simulink model "nonlinear_system"  (R2023b)
settings: Solver=VariableStepAuto  StartTime=0.0  StopTime=10  RelTol=1e-3
values from neighbouring files (symbols this model uses):
  Bl = 0    [collaborative_class_main.m]    (also in n0_collaborative_class_main.m; svc_robot.m)
  Bm = 0.015    [collaborative_class_main.m]    (also in n0_collaborative_class_main.m; svc_robot.m)
  g = 9.81    [collaborative_class_main.m]    (also in n0_collaborative_class_main.m; svc_robot.m)
  Jl = 4e-4    (= 0.0004)    [collaborative_class_main.m]    (also in n0_collaborative_class_main.m; svc_robot.m)
  Jm = 4e-4    (= 0.0004)    [collaborative_class_main.m]    (also in n0_collaborative_class_main.m; svc_robot.m)
  k = 0.8    [collaborative_class_main.m]    (also in n0_collaborative_class_main.m; svc_robot.m)
  K_lqeta = K_lqe(:, 5)    [collaborative_class_main.m]    (also in n0_collaborative_class_main.m = K_lq_ext(:,5))
  K_lqx = K_lqe(:,1:4)    [collaborative_class_main.m]    (also in n0_collaborative_class_main.m = K_lq_ext(:,1:4))
  Kv = -K_ext(1, 5)    [collaborative_class_main.m]    (also in n0_collaborative_class_main.m)
  Kx = -K_ext(1, 1:4)    [collaborative_class_main.m]    (also in n0_collaborative_class_main.m)
  l = 0.3    [collaborative_class_main.m]    (also in n0_collaborative_class_main.m; svc_robot.m)
  m = 0.3    [collaborative_class_main.m]    (also in n0_collaborative_class_main.m; svc_robot.m)
  u_bar = m*g*l*cos(x2_bar)    [collaborative_class_main.m]    (also in n0_collaborative_class_main.m; svc_robot.m)
  x_0 = x_bar+0.01    [collaborative_class_main.m]
  x_bar = [x1_bar x2_bar x3_bar x4_bar]    [collaborative_class_main.m]    (also in n0_collaborative_class_main.m; svc_robot.m = [x1_bar x2_bar x3_bar x4_bar]')
settings Model: Creator=alexz  LastModifiedBy=teoma

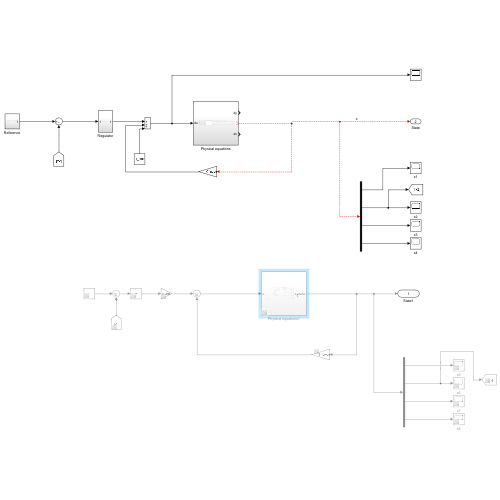
[thumbnail: Simulink's stored preview of the top-level diagram]
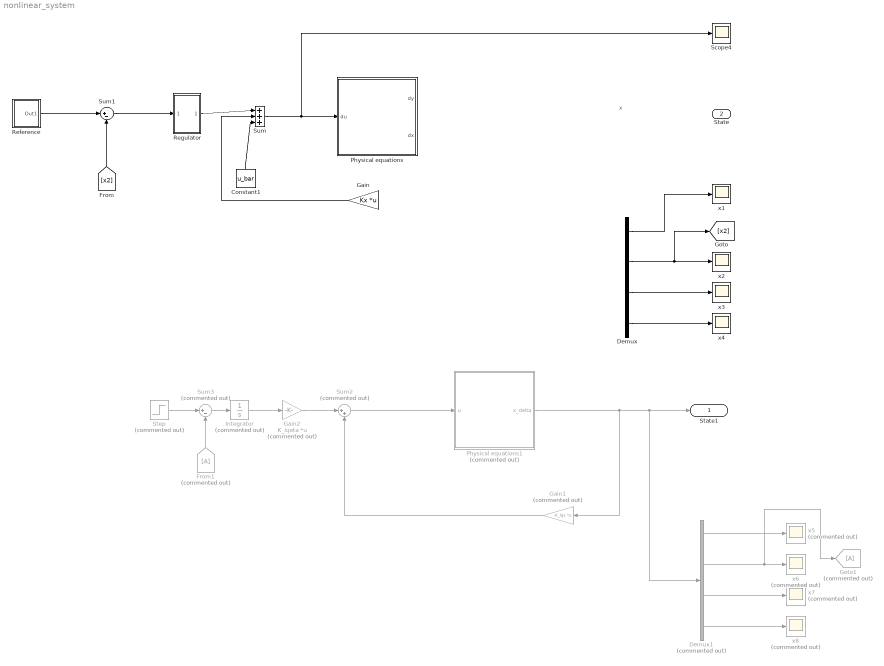
== system nonlinear_system ==
  note: x
  Constant1 : Constant  Value=u_bar
  Demux : Demux
  Demux1 : Demux  Commented=on
  From1 : From  Commented=on
  Gain : Gain  Gain=Kx  Multiplication=Matrix(K*u) (u vector)
  Gain1 : Gain  Commented=on  Gain=-K_lqx  Multiplication=Matrix(K*u) (u vector)
  Gain2 : Gain  Commented=on  Gain=K_lqeta  Multiplication=Matrix(K*u) (u vector)
  Goto1 : Goto  Commented=on
  Integrator : Integrator  Commented=on
  Physical equations : Subsystem
  Physical equations1 : Subsystem  Commented=on
  Reference : Subsystem
  Regulator : Subsystem
  Scope4 : Scope
  Step : Step  Commented=on  SampleTime=0
  Sum : Sum  Inputs=|+++
  Sum1 : Sum  Inputs=|+-
  Sum2 : Sum  Commented=on  Inputs=|++
  Sum3 : Sum  Commented=on  Inputs=|+-
  x{1..4} (4 alike) : Scope
  x{5..8} (4 alike) : Scope  Commented=on
  State1 : Outport
  State : Outport  Port=2
  wires:
  Sum1/1 -> Regulator/1(In1)
  [x2] -> Sum1/2
  Regulator/1(Out1) -> Sum/1
  ? -> Demux/1, State/1, Gain/1
  Gain/1 -> Sum/2
  Sum/1 -> Physical equations/1(du), Scope4/1
  Demux/1 -> x1/1
  Demux/4 -> x4/1
  Demux/3 -> x3/1
  Demux/2 -> [x2], x2/1
  Reference/1(Out1) -> Sum1/1
  Constant1/1 -> Sum/3
  Physical equations1/1(x_delta) -> Gain1/1, Demux1/1, State1/1
  Sum2/1 -> Physical equations1/1(u)
  Gain1/1 -> Sum2/2
  Demux1/1 -> x5/1
  Demux1/4 -> x8/1
  Demux1/3 -> x7/1
  Demux1/2 -> Goto1/1, x6/1
  Sum3/1 -> Integrator/1
  From1/1 -> Sum3/2
  Gain2/1 -> Sum2/1
  Integrator/1 -> Gain2/1
  Step/1 -> Sum3/1

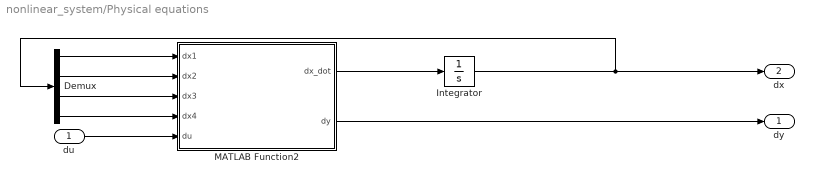
== system nonlinear_system/Physical equations ==
  du : Inport
  Demux : Demux
  Integrator : Integrator  InitialCondition=[0;0;0;0]+1
  MATLAB Function2 : MATLAB Function  TreatAsAtomicUnit=on
  dy : Outport
  dx : Outport  Port=2
  wires:
  MATLAB Function2/2(dy) -> dy/1
  MATLAB Function2/1(dx_dot) -> Integrator/1
  du/1 -> MATLAB Function2/5(du)
  Demux/3 -> MATLAB Function2/3(dx3)
  Demux/2 -> MATLAB Function2/2(dx2)
  Demux/1 -> MATLAB Function2/1(dx1)
  Integrator/1 -> Demux/1, dx/1
  Demux/4 -> MATLAB Function2/4(dx4)

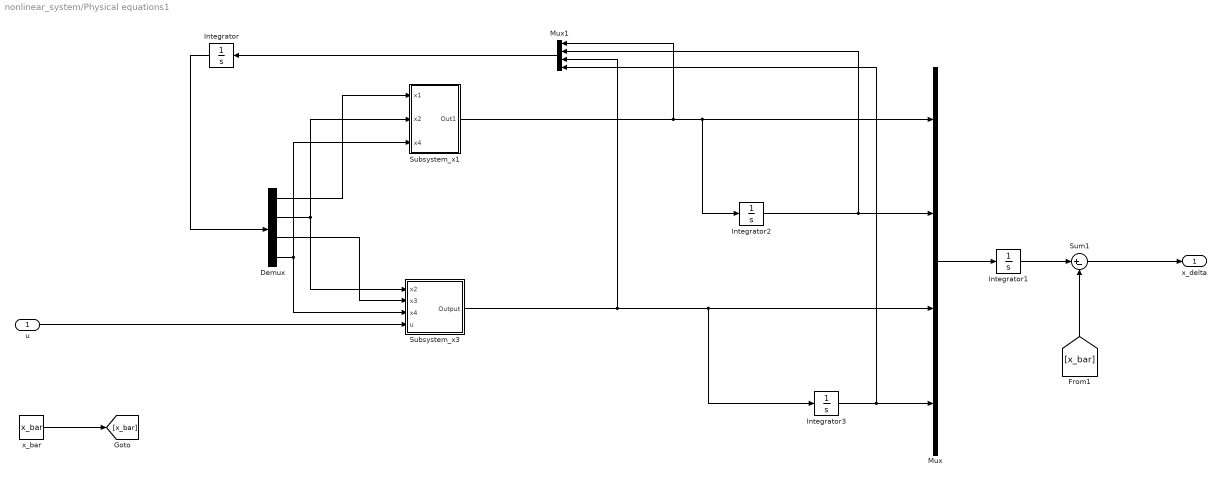
== system nonlinear_system/Physical equations1 ==
  u : Inport
  Demux : Demux
  Integrator : Integrator  InitialCondition=x_0
  Integrator1 : Integrator
  Integrator2 : Integrator
  Integrator3 : Integrator
  Mux : Mux
  Mux1 : Mux
  Subsystem_x1 : Subsystem
  Subsystem_x3 : Subsystem
  Sum1 : Sum  Inputs=|+-
  x_bar : Constant  Value=x_bar
  x_delta : Outport
  wires:
  u/1 -> Subsystem_x3/4(u)
  Integrator/1 -> Demux/1
  x_bar/1 -> [x_bar]
  Mux1/1 -> Integrator/1
  Mux/1 -> Integrator1/1
  Demux/1 -> Subsystem_x1/1(x1)
  Demux/2 -> Subsystem_x3/1(x2), Subsystem_x1/2(x2)
  Demux/3 -> Subsystem_x3/2(x3)
  Subsystem_x3/1(Output) -> Mux1/3, Integrator3/1, Mux/3
  Demux/4 -> Subsystem_x3/3(x4), Subsystem_x1/3(x4)
  Subsystem_x1/1(Out1) -> Mux1/1, Integrator2/1, Mux/1
  Integrator2/1 -> Mux1/2, Mux/2
  Integrator3/1 -> Mux1/4, Mux/4
  [x_bar] -> Sum1/2
  Integrator1/1 -> Sum1/1
  Sum1/1 -> x_delta/1

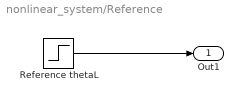
== system nonlinear_system/Reference ==
  Reference thetaL : Step  After=pi/4  SampleTime=0
  Out1 : Outport
  wires:
  Reference thetaL/1 -> Out1/1

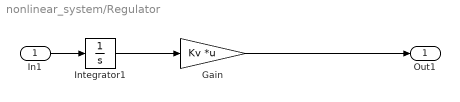
== system nonlinear_system/Regulator ==
  In1 : Inport
  Gain : Gain  Gain=Kv  Multiplication=Matrix(K*u) (u vector)
  Integrator1 : Integrator
  Out1 : Outport
  wires:
  In1/1 -> Integrator1/1
  Gain/1 -> Out1/1
  Integrator1/1 -> Gain/1

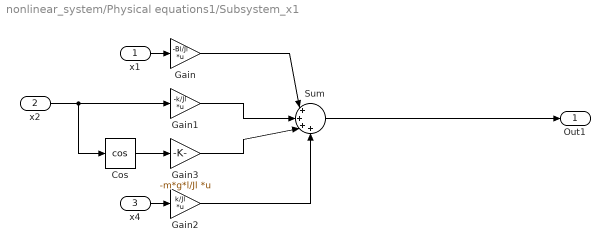
== system nonlinear_system/Physical equations1/Subsystem_x1 ==
  x1 : Inport
  x2 : Inport  Port=2
  x4 : Inport  Port=3
  Cos : Trigonometry  Operator=cos
  Gain : Gain  Gain=-Bl/Jl  Multiplication=Matrix(K*u) (u vector)
  Gain1 : Gain  Gain=-k/Jl  Multiplication=Matrix(K*u) (u vector)
  Gain2 : Gain  Gain=k/Jl  Multiplication=Matrix(K*u) (u vector)
  Gain3 : Gain  Gain=-m*g*l/Jl  Multiplication=Matrix(K*u) (u vector)
  Sum : Sum  Inputs=|++++
  Out1 : Outport
  wires:
  x1/1 -> Gain/1
  Gain3/1 -> Sum/3
  Gain1/1 -> Sum/2
  Gain/1 -> Sum/1
  Cos/1 -> Gain3/1
  Gain2/1 -> Sum/4
  Sum/1 -> Out1/1
  x4/1 -> Gain2/1
  x2/1 -> Cos/1, Gain1/1

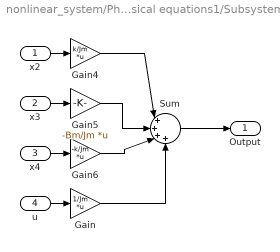
== system nonlinear_system/Physical equations1/Subsystem_x3 ==
  x2 : Inport
  x3 : Inport  Port=2
  x4 : Inport  Port=3
  u : Inport  Port=4
  Gain : Gain  Gain=1/Jm  Multiplication=Matrix(K*u) (u vector)
  Gain4 : Gain  Gain=k/Jm  Multiplication=Matrix(K*u) (u vector)
  Gain5 : Gain  Gain=-Bm/Jm  Multiplication=Matrix(K*u) (u vector)
  Gain6 : Gain  Gain=-k/Jm  Multiplication=Matrix(K*u) (u vector)
  Sum : Sum  Inputs=|++++
  Output : Outport
  wires:
  x2/1 -> Gain4/1
  x4/1 -> Gain6/1
  x3/1 -> Gain5/1
  u/1 -> Gain/1
  Gain4/1 -> Sum/1
  Gain5/1 -> Sum/2
  Gain6/1 -> Sum/3
  Gain/1 -> Sum/4
  Sum/1 -> Output/1

== matlab function nonlinear_system/Physical equations/MATLAB Function2 ==
  data: dx1 input; dx2 input; dx3 input; dx4 input; du input; dx_dot output; dy output
function [dx_dot, dy]  = fcn(dx1,dx2,dx3,dx4, du)

k = 0.8;
Jm = 4e-4;
Jl= 4e-4;
Bm = 0.015;
Bl = 0;
m = 0.3;
l = 0.3;
g = 9.81;
x1_bar = 0;
x2_bar = pi/4;
x3_bar = 0;
x4_bar = m*g*l*cos(x2_bar)/k + x2_bar;
u_bar= m*g*l*cos(x2_bar);


dx1_dot = -k/Jl*(dx2+x2_bar)-m*g*l/Jl*(cos(dx2+x2_bar))+k/Jl*(dx4+x4_bar);
dx2_dot = dx1+x1_bar;
dx3_dot = k/Jm*(dx2+x2_bar)-Bm/Jm*(dx3+x3_bar)-k/Jm*(dx4+x4_bar)+1/Jm*(du+u_bar);
dx4_dot = dx3+x3_bar;
dy = pi/4 - (dx2+x2_bar);

dx_dot = zeros(1,4);
dx_dot(1) = dx1_dot;
dx_dot(2) = dx2_dot;
dx_dot(3) = dx3_dot;
dx_dot(4) = dx4_dot;
